simulink model "simulinkPBLextended"  (R2020b)
settings: Solver=VariableStepAuto  StartTime=0.0  StopTime=100000  RelTol=1e-3
model workspace (MAT data in the model file):
  ON_OFF = 0
  SL_ROS_VariableLengthArrays_MaxSizes : object (value not decoded)
values from neighbouring files (symbols this model uses):
  distToReach = 0.1    [scriptPBLextended.m]
  mapSize = zeros(7,7)    [scriptPBLextended.m]
  myGoals = [  2.5   1  1;                0.2   1   0]    [scriptPBLextended.m]
  slow_ang = 0.2    [scriptPBLextended.m]
  slow_vel = 0.2    [scriptPBLextended.m]
  vizLim = [5;5;0;0]    [scriptPBLextended.m]
undefined symbols (not defined in the file or in its folder): Angular, Linear
libraries: robotlib x9, robotalgslib x2, robotcorelib x1
(part 3 of 3)

== system simulinkPBLextended/Arm Communication/Subsystem ==
  steering v2 : Inport
  Clock : Clock
  Constant : Constant  Value=false
  Constant1 : Constant  Value=0
  Constant2 : Constant  Value=true
  MATLAB Function2 : MATLAB Function  TreatAsAtomicUnit=on
  Switch : Switch  Threshold=1
  Switch1 : Switch  Criteria=u2 > Threshold  Threshold=2
  Out1 : Outport
  wires:
  Constant/1 -> Switch1/3
  steering v2/1 -> Switch1/1
  Clock/1 -> Switch1/2
  Switch/1 -> Out1/1
  Constant1/1 -> Switch/2
  Constant2/1 -> Switch/1
  Switch1/1 -> MATLAB Function2/1(u)
  MATLAB Function2/1(y) -> Switch/3

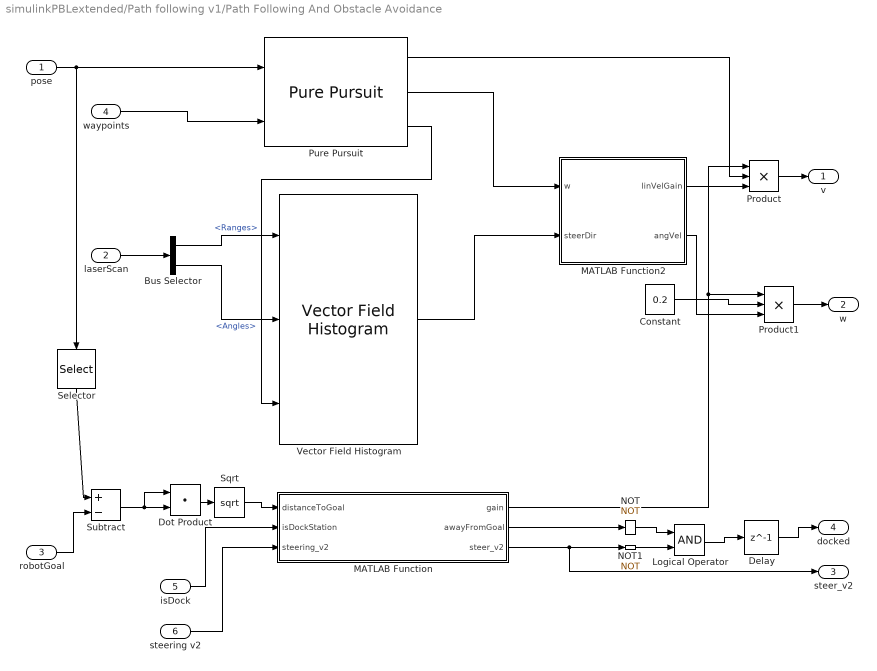
== system simulinkPBLextended/Path following v1/Path Following And Obstacle Avoidance ==
  pose : Inport
  laserScan : Inport  Port=2
  robotGoal : Inport  Port=3
  waypoints : Inport  Port=4
  isDock : Inport  Port=5
  steering v2 : Inport  Port=6
  Bus Selector : BusSelector  OutputSignals=Ranges,Angles
  Constant : Constant  Value=0.2
  Delay : Delay  DelayLength=1  InitialCondition=0
  Dot Product : DotProduct  InputSameDT=on  OutDataTypeStr=Inherit: Inherit via internal rule
  Logical Operator : Logic  AllPortsSameDT=off  OutDataTypeStr=boolean
  MATLAB Function : MATLAB Function  TreatAsAtomicUnit=on
  MATLAB Function2 : MATLAB Function  TreatAsAtomicUnit=on
  NOT : Logic  Operator=NOT  AllPortsSameDT=off  OutDataTypeStr=boolean
  NOT1 : Logic  Operator=NOT  AllPortsSameDT=off  OutDataTypeStr=boolean
  Product : Product  Inputs=3
  Product1 : Product  Inputs=3
  Pure Pursuit : robotalgslib/Pure Pursuit  DesiredLinearVelocity=desired_vel  MaxAngularVelocity=max_ang_vel  LookaheadDistance=2  TargetDirPort=on  SimulateUsing=Code generation
  Selector : Selector  InputPortWidth=3  IndexOptions=Index vector (dialog)  Indices=[1 2]  OutputSizes=1
  Sqrt : Sqrt  SaturateOnIntegerOverflow=on
  Subtract : Sum  Inputs=+-
  Vector Field Histogram : robotalgslib/Vector Field Histogram  NumAngularSectors=180  DistanceLimits=[ 0.02, 3]  HistogramThresholds=[ 3, 10 ]  RobotRadius=0.1  SafetyDistance=0  MinTurningRadius=1  SimulateUsing=Code generation  TargetDirectionWeight=3  CurrentDirectionWeight=0.5  PreviousDirectionWeight=2
      settings: SourceProductBaseCode=NV,RO
  v : Outport
  w : Outport  Port=2
  steer_v2 : Outport  Port=3
  docked : Outport  Port=4
  wires:
  Pure Pursuit/1 -> Product/2
  MATLAB Function/1(gain) -> Product/1, Product1/1
  laserScan/1 -> Bus Selector/1
  Sqrt/1 -> MATLAB Function/1(distanceToGoal)
  Subtract/1 -> Dot Product/1, Dot Product/2
  Selector/1 -> Subtract/1
  Dot Product/1 -> Sqrt/1
  robotGoal/1 -> Subtract/2
  pose/1 -> Selector/1, Pure Pursuit/1
  waypoints/1 -> Pure Pursuit/2
  Bus Selector/2 -> Vector Field Histogram/2  "<Angles>"
  Bus Selector/1 -> Vector Field Histogram/1  "<Ranges>"
  Product1/1 -> w/1
  Product/1 -> v/1
  Pure Pursuit/3 -> Vector Field Histogram/3
  Vector Field Histogram/1 -> MATLAB Function2/2(steerDir)
  Pure Pursuit/2 -> MATLAB Function2/1(w)
  MATLAB Function2/1(linVelGain) -> Product/3
  MATLAB Function2/2(angVel) -> Product1/3
  isDock/1 -> MATLAB Function/2(isDockStation)
  steering v2/1 -> MATLAB Function/3(steering_v2)
  MATLAB Function/3(steer_v2) -> steer_v2/1, NOT1/1
  Logical Operator/1 -> Delay/1
  MATLAB Function/2(awayFromGoal) -> NOT/1
  NOT/1 -> Logical Operator/1
  NOT1/1 -> Logical Operator/2
  Delay/1 -> docked/1
  Constant/1 -> Product1/2

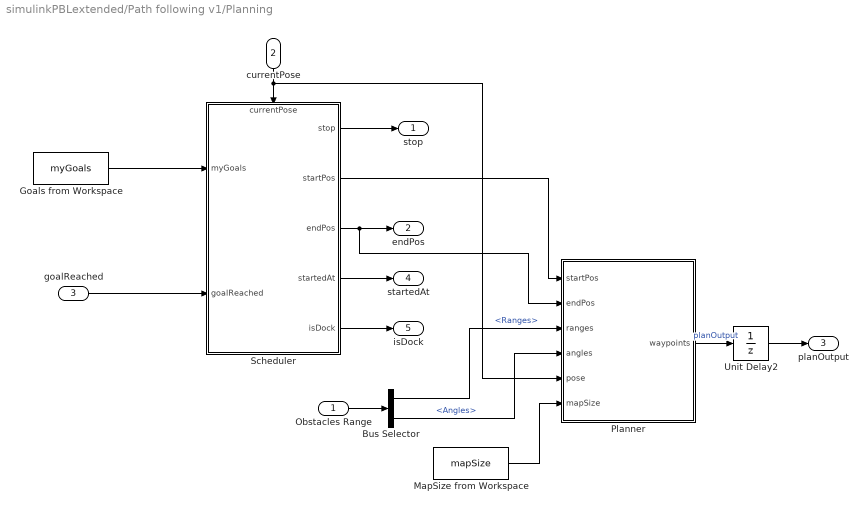
== system simulinkPBLextended/Path following v1/Planning ==
  Obstacles Range : Inport
  currentPose : Inport  Port=2
  goalReached : Inport  Port=3
  Bus Selector : BusSelector  OutputSignals=Ranges,Angles
  "Goals from Workspace " : Constant  Value=myGoals  SampleTime=1
  MapSize from Workspace : Constant  Value=mapSize  SampleTime=1
  Planner : MATLAB Function  TreatAsAtomicUnit=on
  Scheduler : Stateflow chart  TreatAsAtomicUnit=on
      settings: PortSchema="{\"entries\":[{\"content\":{\"sides\":[{\"content\":{\"connectorIds\":[\"In2\",\"In3\"]},\"type\":\"ConnectorPlacement.EquallySpacedRectSide\",\"uuid\":\"99158a3b-161c-4263-a7f9-9d21b7748630\"},{\"content\":{\"connectorIds\":[\"Out1\",\"Out2\",\"Out3\",\"Out4\",\"Out5\"],\"side\":\"RIGHT\"},\"type\":\"ConnectorPlacement.EquallySpacedRectSide\",\"uuid\":\"468729f6-200a-43c1-864b-c0af8f1f8d51\"},{\"content\":{\"connectorIds\":[\"In1\"],\"side\":\"TOP\"},\"type\":\"ConnectorPlacement.EquallySpacedRectSide\",\"uuid\":\"3b2da12a-8f16-4687-80ee-3d598f82b8bb\"},{\"content\":{\"connectorIds\":[],\"side\":\"HIDDEN\"},\"type\":\"ConnectorPlacement.EquallySpacedRectSide\",\"uuid\":\"e29f059b-8c47-4618-8070-0e514e32b359\"}]},\"type\":\"ConnectorPlacement.EquallySpacedConnector\",\"uuid\":\"701eb0d1-f061-4bcf-9183-74b290beee5f\"}],\"packageUris\":[\"http://schema.mathworks.com/mf0/Connector/R2020b\"],\"version\":\"1.0\"}"
  Unit Delay2 : UnitDelay  SampleTime=-1  HasFrameUpgradeWarning=on
  stop : Outport
  endPos : Outport  Port=2
  planOutput : Outport  Port=3
  startedAt : Outport  Port=4
  isDock : Outport  Port=5
  wires:
  "Goals from Workspace "/1 -> Scheduler/2(myGoals)
  Scheduler/1(stop) -> stop/1
  Scheduler/2(startPos) -> Planner/1(startPos)
  goalReached/1 -> Scheduler/3(goalReached)
  Scheduler/3(endPos) -> Planner/2(endPos), endPos/1
  currentPose/1 -> Planner/5(pose), Scheduler/1(currentPose)
  Obstacles Range/1 -> Bus Selector/1
  Bus Selector/1 -> Planner/3(ranges)  "<Ranges>"
  Bus Selector/2 -> Planner/4(angles)  "<Angles>"
  Scheduler/4(startedAt) -> startedAt/1
  MapSize from Workspace/1 -> Planner/6(mapSize)
  Planner/1(waypoints) -> Unit Delay2/1  "planOutput"
  Unit Delay2/1 -> planOutput/1
  Scheduler/5(isDock) -> isDock/1

== system simulinkPBLextended/Path following v2/Enabled Subsystem1 ==
  In1 : Inport
  Enable : EnablePort
  obstaclesRange : Outport
  wires:
  In1/1 -> obstaclesRange/1

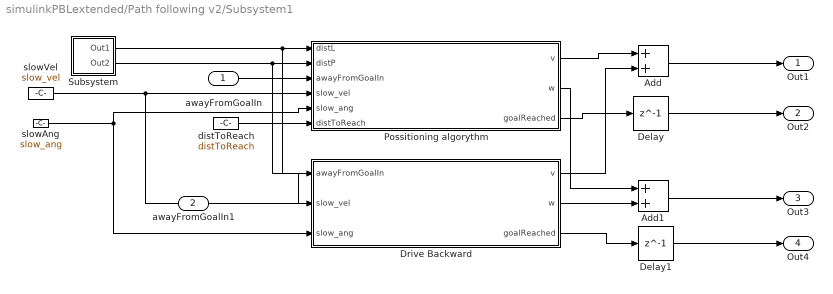
== system simulinkPBLextended/Path following v2/Subsystem1 ==
  awayFromGoalIn : Inport
  awayFromGoalIn1 : Inport  Port=2
  Add : Sum
  Add1 : Sum
  Delay : Delay  DelayLength=1  InitialCondition=0
  Delay1 : Delay  DelayLength=1  InitialCondition=0
  Drive Backward : MATLAB Function  TreatAsAtomicUnit=on
  Possitioning algorythm : MATLAB Function  TreatAsAtomicUnit=on
  Subsystem : Subsystem
  distToReach : Constant  Value=distToReach  SampleTime=1
  slowAng : Constant  Value=slow_ang  SampleTime=1
  slowVel : Constant  Value=slow_vel  SampleTime=1
  Out1 : Outport
  Out2 : Outport  Port=2
  Out3 : Outport  Port=3
  Out4 : Outport  Port=4
  wires:
  Drive Backward/3(goalReached) -> Delay1/1
  awayFromGoalIn1/1 -> Drive Backward/1(awayFromGoalIn)
  Drive Backward/2(w) -> Add1/2
  Possitioning algorythm/1(v) -> Add/1
  distToReach/1 -> Possitioning algorythm/6(distToReach)
  Possitioning algorythm/3(goalReached) -> Delay/1
  Delay1/1 -> Out4/1
  Possitioning algorythm/2(w) -> Add1/1
  Add1/1 -> Out3/1
  slowVel/1 -> Drive Backward/2(slow_vel), Possitioning algorythm/4(slow_vel)
  Delay/1 -> Out2/1
  slowAng/1 -> Possitioning algorythm/5(slow_ang), Drive Backward/3(slow_ang)
  Drive Backward/1(v) -> Add/2
  Add/1 -> Out1/1
  awayFromGoalIn/1 -> Possitioning algorythm/3(awayFromGoalIn)
  Subsystem/2(Out2) -> Possitioning algorythm/2(distP)
  Subsystem/1(Out1) -> Possitioning algorythm/1(distL)

== system simulinkPBLextended/Pioneer Wheel Control/Subsystem ==
  In1 : Inport
  Clock : Clock
  Constant : Constant  Value=0
  Switch1 : Switch  Criteria=u2 > Threshold  Threshold=2
  Out1 : Outport
  wires:
  Switch1/1 -> Out1/1
  Constant/1 -> Switch1/3
  In1/1 -> Switch1/1
  Clock/1 -> Switch1/2

== system simulinkPBLextended/Pioneer Wheel Control/Subsystem1 ==
  w : Inport
  Clock : Clock
  Constant : Constant  Value=0
  Switch1 : Switch  Criteria=u2 > Threshold  Threshold=2
  Out1 : Outport
  wires:
  Switch1/1 -> Out1/1
  Constant/1 -> Switch1/3
  w/1 -> Switch1/1
  Clock/1 -> Switch1/2

== system simulinkPBLextended/ROS Subscribers/Enabled Subsystem1 ==
  In1 : Inport
  Enable : EnablePort
  obstaclesRange : Outport
  wires:
  In1/1 -> obstaclesRange/1

== system simulinkPBLextended/ROS Subscribers/Enabled Subsystem2 ==
  In1 : Inport
  Enable : EnablePort
  Bus Selector1 : BusSelector  OutputSignals=Data
  obstaclesRange : Outport
  wires:
  In1/1 -> Bus Selector1/1
  Bus Selector1/1 -> obstaclesRange/1  "<Data>"

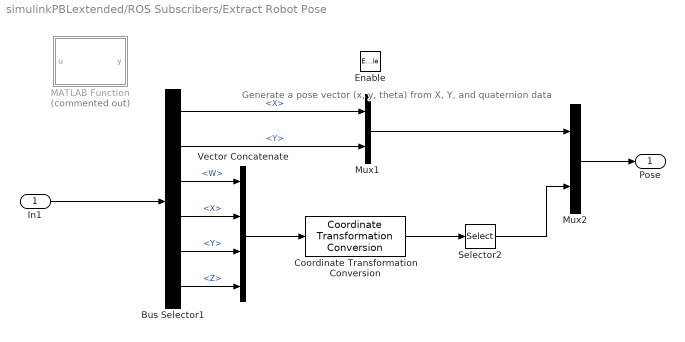
== system simulinkPBLextended/ROS Subscribers/Extract Robot Pose ==
  note: Generate a pose vector (x, y, theta) from X, Y, and quaternion data
  In1 : Inport
  Enable : EnablePort
  Bus Selector1 : BusSelector  OutputSignals=Pose.Pose.Position.X,Pose.Pose.Position.Y,Pose.Pose.Orientation.W,Pose.Pose.Orientation.X,Pose.Pose.Orientation.Y,Pose.Pose.Orientation.Z
  Coordinate Transformation Conversion : robotcorelib/Coordinate Transformation Conversion  InputRepresentation=Quaternion  InputEulerSequence=ZYX  ShowTrVecInputPort=on  OutputRepresentation=Euler Angles  OutputEulerSequence=ZYX  ShowTrVecOutputPort=on  SimulateUsing=Interpreted execution
  MATLAB Function : MATLAB Function  Commented=on  TreatAsAtomicUnit=on
  Mux1 : Mux  Inputs=2
  Mux2 : Mux  Inputs=2
  Selector2 : Selector  InputPortWidth=3  IndexOptions=Index vector (dialog)  Indices=1  OutputSizes=1
  Vector Concatenate : Concatenate  NumInputs=4
  Pose : Outport  VectorParamsAs1DForOutWhenUnconnected=off
  wires:
  Vector Concatenate/1 -> Coordinate Transformation Conversion/1
  Coordinate Transformation Conversion/1 -> Selector2/1
  Mux1/1 -> Mux2/1
  Selector2/1 -> Mux2/2
  Mux2/1 -> Pose/1
  Bus Selector1/4 -> Vector Concatenate/2  "<X>"
  Bus Selector1/6 -> Vector Concatenate/4  "<Z>"
  Bus Selector1/2 -> Mux1/2  "<Y>"
  Bus Selector1/3 -> Vector Concatenate/1  "<W>"
  Bus Selector1/5 -> Vector Concatenate/3  "<Y>"
  In1/1 -> Bus Selector1/1
  Bus Selector1/1 -> Mux1/1  "<X>"

== system simulinkPBLextended/ROS Subscribers/Subsystem ==
  In1 : Inport
  Constant3 : Constant  Value=0
  Constant6 : Constant  Value=true
  MATLAB Function2 : MATLAB Function  TreatAsAtomicUnit=on
  Switch3 : Switch  Threshold=1
  y : Outport
  wires:
  Switch3/1 -> MATLAB Function2/1(u)
  Constant3/1 -> Switch3/2
  MATLAB Function2/1(y) -> y/1
  In1/1 -> Switch3/3
  Constant6/1 -> Switch3/1

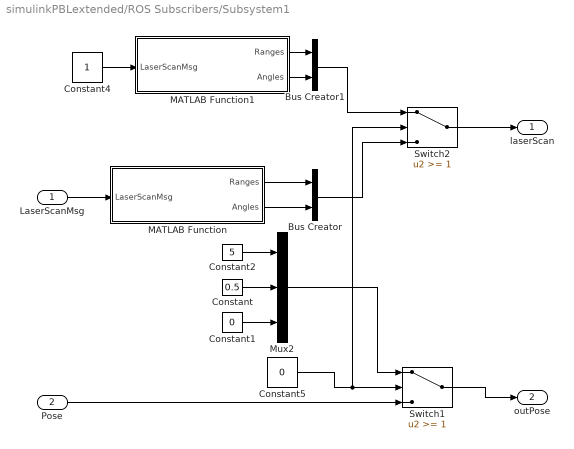
== system simulinkPBLextended/ROS Subscribers/Subsystem1 ==
  LaserScanMsg : Inport
  Pose : Inport  Port=2
  Bus Creator : BusCreator  Inputs=2
  Bus Creator1 : BusCreator  Inputs=2
  Constant : Constant  Value=0.5
  Constant1 : Constant  Value=0
  Constant2 : Constant  Value=5
  Constant4 : Constant
  Constant5 : Constant  Value=0
  MATLAB Function : MATLAB Function  TreatAsAtomicUnit=on
  MATLAB Function1 : MATLAB Function  TreatAsAtomicUnit=on
  Mux2 : Mux  Inputs=3
  Switch1 : Switch  Threshold=1
  Switch2 : Switch  Threshold=1
  laserScan : Outport
  outPose : Outport  Port=2
  wires:
  Pose/1 -> Switch1/3
  Constant5/1 -> Switch2/2, Switch1/2
  MATLAB Function/2(Angles) -> Bus Creator/2
  Mux2/1 -> Switch1/1
  Constant2/1 -> Mux2/1
  MATLAB Function/1(Ranges) -> Bus Creator/1
  Switch1/1 -> outPose/1
  Bus Creator/1 -> Switch2/3
  Bus Creator1/1 -> Switch2/1
  LaserScanMsg/1 -> MATLAB Function/1(LaserScanMsg)
  MATLAB Function1/1(Ranges) -> Bus Creator1/1
  Constant4/1 -> MATLAB Function1/1(LaserScanMsg)
  Constant1/1 -> Mux2/3
  Switch2/1 -> laserScan/1
  MATLAB Function1/2(Angles) -> Bus Creator1/2
  Constant/1 -> Mux2/2

== system simulinkPBLextended/Path following v2/Subsystem1/Subsystem ==
  Bus Selector1 : BusSelector  OutputSignals=Echoes
  Constant : Constant
  Constant1 : Constant  Value=0
  Enabled Subsystem2 : Subsystem  TreatAsAtomicUnit=on
  Subscribe1 : robotlib/Subscribe  topicSource=Specify your own  topic=/robot_driver/laser_ruler/scan  messageType=sensor_msgs/LaserEcho  SampleTime=-1  legacyBusStruct=off  messageQueueLength=1
  Switch1 : Switch  Threshold=1
  Switch2 : Switch  Threshold=1
  Out1 : Outport
  Out2 : Outport  Port=2
  wires:
  Subscribe1/1 -> Enabled Subsystem2/Enable
  Bus Selector1/1 -> Enabled Subsystem2/1(LaserScanMsg)  "<Echoes>"
  Constant1/1 -> Switch2/2, Switch1/2
  Switch2/1 -> Out2/1
  Enabled Subsystem2/1(laserPrawy) -> Switch1/3
  Switch1/1 -> Out1/1
  Constant/1 -> Switch2/1, Switch1/1
  Subscribe1/2 -> Bus Selector1/1
  Enabled Subsystem2/2(laserLewy) -> Switch2/3

== system simulinkPBLextended/Path following v2/Subsystem1/Subsystem/Enabled Subsystem2 ==
  LaserScanMsg : Inport
  Enable : EnablePort
  MATLAB Function1 : MATLAB Function  TreatAsAtomicUnit=on
  laserPrawy : Outport
  laserLewy : Outport  Port=2
  wires:
  LaserScanMsg/1 -> MATLAB Function1/1(LaserScanMsg)
  MATLAB Function1/1(laserPrawy) -> laserPrawy/1
  MATLAB Function1/2(laserLewy) -> laserLewy/1

== matlab function simulinkPBLextended/Path following v1/Planning/Planner ==
  settings: updateMethod=DISCRETE
  data: startPos input size=[1 2]; endPos input size=[2 1]; waypoints output size=[200 2]; ranges input; angles input; pose input; mapSize input
function waypoints = planning(startPos, endPos, ranges, angles, pose, mapSize)

persistent waypointsInternal
persistent prevStartPos
persistent prevEndPos
persistent map
    
    maxRange = 10.2;
    resolution = 10;
    xSize=(size(mapSize,1)*10);
    ySize=(size(mapSize,2)*10);

    if isempty(map)
        x=zeros(ySize*2,xSize*2);
        map = occupancyMap(x,resolution);
        map.GridOriginInLocal= [-size(mapSize,1) -size(mapSize,2)];
    end
    
    
    
maxNumNodes = 200;
 
if isempty(prevStartPos)
    prevStartPos = startPos;
end

if isempty(prevEndPos)
    prevEndPos = endPos;
end

    
isNewPath = (~isequal(prevStartPos, startPos) || ~isequal(prevEndPos, endPos));

% Dwa warunki, w których muszą być ustawione punkty trasy: nie są 
% jeszcze zainicjowane lub są zainicjowane, ale bieżący początek i koniec 
% nie odpowiadają tym, które zostały użyte do wygenerowania poprzedniego 
% zestawu punktów trasy.
if isempty(waypointsInternal) || isNewPath
    startPosition= pose(1:2)';
    %plan path to funkcja zaimplementowana ponizej
    [waypointsInternal] = planPath(map, maxNumNodes, startPosition, endPos);
end

    if ~isempty(ranges)
            characterPose = [pose(1) pose(2) pose(3)];
            insertRay(map, characterPose, ranges, angles, maxRange);
    end
% Aktualizacja wyników punktow trasy
waypoints = waypointsInternal;

% Aktualizacja zmiennych trwałych wskazujących poprzedni stan
prevStartPos = startPos;
prevEndPos = endPos;

%% Funkcja pomocnicza do planowania trasy
function wayPoints = planPath(map, maxNodes, startPos, endPos)
    
    % Utworzenie "mapy drog"
    prm = mobileRobotPRM(map, maxNodes);
%     prm.ConnectionDistance=5;
    
    % Znalezienie najlepszej sciezki pomiedzy punktem startu i koncowym
    xy = findpath(prm, startPos(:)', endPos(:)');
    wayPoints = repmat(endPos(:)', maxNodes, 1);
    
    % Liczba węzłów, które są faktycznie wykorzystywane
    numNodes = length(xy);
    wayPoints(1:numNodes,:) = xy; 
    
    
end

end

== matlab function simulinkPBLextended/Path following v1/Path Following And Obstacle Avoidance/MATLAB Function2 ==
  data: linVelGain output; w input; steerDir input; angVel output
function [linVelGain, angVel]= steer(w, steerDir)
%steer Outputs the angular velocity corresponding to the steering direction
%   If a steering direction is provided, steer the robot in that direction,
%   else continue with the angular velocity that the robot was already
%   pursuing.
linVelGain = 1;
if(~isnan(steerDir) && abs(steerDir)) 
    angVel = steerDir;
    linVelGain = 1;
else
    angVel = w;
end

== stateflow chart simulinkPBLextended/Path following v1/Planning/Scheduler ==
  settings: sampleTime=0.01
  state MyGoal
    entry:
    if(i>size(myGoals,1))
    stop=true;
    else
    if(myGoals(i,3))
    isDock=true;
    else
    isDock=false;
    end
    endPos = myGoals(i,1:2)';
    end
    during:
    endPos = myGoals(i,1:2)';
    exit:
    i = i + 1;
  state MyAnotherGoal
    entry:
    if(i>size(myGoals,1))
    stop=true;
    else
    if(myGoals(i,3))
    isDock=true;
    else
    isDock=false;
    end
    endPos = myGoals(i,1:2)';
    end
    during:
    endPos = myGoals(i,1:2)';
    exit:
    i = i + 1;
  (default) -> MyGoal : {startPos = currentPose(1:2)';
      |  i=1;
      |  startedAt = currentPose(1:2)';}
  MyGoal -> MyAnotherGoal : [goalReached==1]
      | {startPos = currentPose(1:2)';}
  MyAnotherGoal -> MyGoal : [goalReached==1]
      | {startPos = currentPose(1:2)';}
  data: currentPose input; stop output boolean =false; myGoals input; startPos output size=[1, 2]; endPos output size=[2, 1]; goalReached input; i local; startedAt output; isDock output

== matlab function simulinkPBLextended/Visualize Robot/Visualization ==
  data: showViz input; robotPoses input; wayPoints input; ranges input; angles input; showPaths input; xLim input; yLim input; MeshSelectionIdx parameter; GoalStation input; StartLocation input; vizLim input
function simulationVisualization(showViz, robotPoses, wayPoints, ranges, angles, showPaths, xLim, yLim, MeshSelectionIdx, GoalStation, StartLocation, vizLim)
%#codegen
 if(robotPoses(1,:)>yLim(2))
     robotPoses(1,:)=yLim(2);
 elseif(robotPoses(1,:)<yLim(1))
     robotPoses(1,:)=yLim(1);
 end
 if(robotPoses(2,:)>xLim(2))
     robotPoses(2,:)=xLim(2);
 elseif(robotPoses(2,:)<xLim(1))
     robotPoses(2,:)=xLim(1);
 end
 
%% Setup
coder.extrinsic('helperVisualizeExecuteRobots');
persistent f
if isempty(f) && showViz
    f = figure('units','normalized','outerposition',[0 0 0.75 0.75]);
    title('Mobile Robot Motion');
    set(f, 'Visible', 'on');
end

% Robot mesh options are cells of the unloaded and loaded robot mesh and
% the translation between the visualized origin and the desired origin
% meshOptions = {...
%     {'groundvehicle.stl', [.314 0 .155], 'groundvehiclewithload.stl', [.312 0 .156]}, ...
%     {'forkliftExecuteRobotTasks.stl', [.3569 0 .297], 'forkliftwithload.stl', [.3813 0 .2893]}, ...
%     };

meshOptions = {...
    {'groundvehicle.stl', [.157 0 .0775], 'groundvehiclewithload.stl', [.156 0 .078]}, ...
    {'forkliftExecuteRobotTasks.stl', [.3569 0 .297], 'forkliftwithload.stl', [.3813 0 .2893]}, ...
    };


if showViz && ~isempty(f)
    helperVisualizeExecuteRobots(f, robotPoses, wayPoints, ranges, angles, StartLocation, GoalStation, showPaths, xLim, yLim, meshOptions{MeshSelectionIdx},vizLim);
end
end

== matlab function simulinkPBLextended/ROS Subscribers/Subsystem1/MATLAB Function ==
  data: LaserScanMsg input; Ranges output; Angles output
function [Ranges, Angles] = ExtractRangeData(LaserScanMsg)
 
% samples=360;
% Ekstrakcja informacji o zasiegu
% Ranges = double(LaserScanMsg.Ranges(1:samples));
Ranges = double(LaserScanMsg.Ranges);
% Skonstruuj wektor kątów używając AngleMin i AngleIncrement z odczytu
% czujnika
angMin = double(LaserScanMsg.AngleMin+(3.14));
angIncrement = double(LaserScanMsg.AngleIncrement);

numReadings = numel(Ranges);

rawAngles = angMin + (0:numReadings-1)' * angIncrement;

% Wrap the angles to the (-pi,pi] interval.
Angles = robotics.internal.wrapToPi(double(rawAngles));

== matlab function simulinkPBLextended/Path following v1/Path Following And Obstacle Avoidance/MATLAB Function ==
  data: distanceToGoal input; gain output; awayFromGoal output; steer_v2 output; isDockStation input; steering_v2 input
function [gain, awayFromGoal,steer_v2] = slowDownNearGoal(distanceToGoal,isDockStation, steering_v2)

%% Funkcja stopniowo spowalnia robota, gdy znajdzie sie w poblizu celu
persistent steer;
persistent old_steer;


if(isempty(steer))
    steer= false;
end
if(isempty(old_steer))
    old_steer= false;
end

gain = 1;
awayFromGoal = true;

% if(steer==old_steer)
%     steer=false;
% end


 %Okreslenie w metrach jak daleko od celu powinien zwalniac robot i kiedy
 %powinien sie zatrzymac
atGoalThreshold = 0.3;
wPoblizuCelu= 1.5;
zmianaSterowania = 0.7;

if(steering_v2)
    old_steer=false;
    steer=false;
end

%if the robot is within range and should start slowing down
if((distanceToGoal < wPoblizuCelu) && ~old_steer)
    
    %redukcja predkosci
    gain = 0.7;
    
    if(distanceToGoal < zmianaSterowania)
        if(~isDockStation)
            %od $(zmianaSterowania[m]) od celu jedzie z predkoscia 1/5*VMax
            gain=0.3;
            if(distanceToGoal < atGoalThreshold)
                % Zatrzymuje sie
                gain = 0.0;
                % i wysyla sygnal, ze nalezy sterowac teraz w inny sposob
                awayFromGoal = false;
                steer=false;
            end
        else
                steer=true;
                old_steer=true;
        end
    end
end

if(steer)
    steer_v2=true;
else
    steer_v2=false;
end

if(old_steer)
    gain=0;
end

== matlab function simulinkPBLextended/Path following v2/Subsystem1/Possitioning algorythm ==
  data: distL input; v output; w output; goalReached output; distP input; awayFromGoalIn input; slow_vel input; slow_ang input; distToReach input
function [v, w, goalReached] = algorithm_v2(distL, distP, awayFromGoalIn,slow_vel,slow_ang,distToReach)

persistent startAlgorithm;
persistent stopAlgorithm;
persistent counter;
persistent done;

diffLP = distL-distP;

distLaser=[distL distP];
robotAvgDist= mean(distLaser);

goalReached=false;

w=0;
v=0;

if(~awayFromGoalIn)
    done=false;
end

if(isempty(startAlgorithm))
    startAlgorithm=false;
end

if(isempty(stopAlgorithm))
    stopAlgorithm=false;
end

if(isempty(done))
    done=false;
end

if(isempty(counter))
   counter=0; 
end

if(awayFromGoalIn && ~done)
   startAlgorithm=true;
end

if(startAlgorithm)
    if(distL>0.1 && distP>0.1)
        if(diffLP>0.01)
           v=slow_vel;
           w=0;
        elseif(diffLP<-0.01)
           v=slow_vel;
           w=0;
        else
           v=slow_vel;
           w=0;
        end
    else
        v=0;
        w=0;
        stopAlgorithm=true;
    end
    
    if(stopAlgorithm)
       startAlgorithm=false;
       done=true;
       counter=1;
    end
    
end

if(counter~=0)
    goalReached=true;
    counter=counter+1;
end

if(counter>3)
    counter=0;
end

if(~awayFromGoalIn)
    done=false;
end

end

== matlab function simulinkPBLextended/Path following v2/MATLAB Function ==
  data: LaserScanMsg input; laser_1 output; laser_2 output
function [laser_1, laser_2] = ExtractRangeData(LaserScanMsg)

numLasers=360;
% Ekstrakcja informacji o zasiegu
Ranges = double(LaserScanMsg.Ranges(1:numLasers));

laser_1= Ranges(178);
laser_2= Ranges(182);

== matlab function simulinkPBLextended/ROS Subscribers/Subsystem1/MATLAB Function1 ==
  data: LaserScanMsg input; Ranges output; Angles output
function [Ranges, Angles] = ExtractRangeData(LaserScanMsg)
 
% samples=360;
% Ekstrakcja informacji o zasiegu
% Ranges = double(LaserScanMsg.Ranges(1:samples));
Ranges = 10*ones(1,720);
% Skonstruuj wektor kątów używając AngleMin i AngleIncrement z odczytu
% czujnika
angMin = double(0.01);
angIncrement = double(0.01);

numReadings = numel(Ranges);
rawAngles = angMin + (0:numReadings-1)' * angIncrement;

% Wrap the angles to the (-pi,pi] interval.
Angles =  robotics.internal.wrapToPi(double(rawAngles));

== matlab function simulinkPBLextended/Path following v2/Subsystem1/Subsystem/Enabled Subsystem2/MATLAB Function1 ==
  data: LaserScanMsg input; laserPrawy output size=1; laserLewy output size=1
function [laserPrawy, laserLewy] = ExtractRangeData(LaserScanMsg)

    numLasers=4;

    Ranges = double(LaserScanMsg(1:numLasers));
    for i=1:numLasers
        if(isinf(Ranges(i)))
            Ranges(i)=1;
        end
    end

    laserPrawy= min(Ranges(1),Ranges(2));
    laserLewy= min(Ranges(3),Ranges(4));

== matlab function simulinkPBLextended/ROS Subscribers/Extract Robot Pose/MATLAB Function ==
  data: u input; y output
function y = fcn(u)


y = u + rand(1);

== matlab function simulinkPBLextended/ROS Subscribers/Subsystem/MATLAB Function2 ==
  data: u input; y output
function y = fcn(u)
persistent oldVal

if(isempty(oldVal))
   oldVal=true; 
elseif(~oldVal&&~u)
    oldVal=true;
end

if(isempty(u))
   y=false;
else
   if(oldVal==u)
       y=u;
       oldVal=false;
   else
      y=false;
   end
end

== matlab function simulinkPBLextended/Path following v2/Subsystem1/Drive Backward ==
  data: v output; w output; goalReached output boolean; awayFromGoalIn input; slow_vel input; slow_ang input
function [v, w, goalReached] = algorithm_Out(awayFromGoalIn,slow_vel,slow_ang)

persistent startAlgorithm;
persistent stopAlgorithm;
persistent t;

goalReached=false;

w=0;
v=0;

if(isempty(startAlgorithm))
    startAlgorithm=false;
end

if(isempty(stopAlgorithm))
    stopAlgorithm=false;
end

if(awayFromGoalIn)
   startAlgorithm=true; 
end

if(startAlgorithm)
    if(isempty(t))
        t=tic;
        v=-0.7;
        w=-1;
    elseif(toc(t)<10)
        v=-0.7;
        w=-1;
    else
        stopAlgorithm=true;
    end
    
    if(stopAlgorithm)
       goalReached=true;
       startAlgorithm=false;
       stopAlgorithm=false;
    end
end

end

== matlab function simulinkPBLextended/Arm Communication/Subsystem/MATLAB Function2 ==
  data: u input; y output
function y = fcn(u)
persistent oldVal

if(isempty(oldVal))
   oldVal=true; 
elseif(~oldVal&&~u)
    oldVal=true;
end

if(isempty(u))
   y=false;
else
   if(oldVal==u)
       y=u;
       oldVal=false;
   else
      y=false;
   end
end
